simulink model "Slx001_Examine2_MHMP"  (R2017b)
settings: Solver=FixedStepAuto  StartTime=0.0  StopTime=100  FixedStep=0.1  RelTol=1e-3
libraries: neural x203
(part 3 of 3)

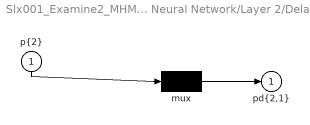
== system Slx001_Examine2_MHMP/Custom Neural Network/Layer 2/Delays 1 ==
  "p{2}" : Inport  PortDimensions=200
      mask Display: e = 0.06;c1 = [120 230 180]/255;c2 = ([120 230 180]+0)/(256+128);c3 = ([120 230 180]+128)/(256+128);patch([0 1 1 0],[0 0 1 1],c1);patch([0 1 1 1-e 1-e 0+e],[0 0 1 1-e 0+e 0+e],c2);patch([0 0 1 1-e 0+e 0+e],[0 1 1 1-e 1-e 0+e],c3);plot([0 1 1 0 0],[0 0 1 1 0]);
  mux : Mux  Inputs=1
      mask Display: e = 0.06;c1 = [120 150 230]/255;c2 = ([120 150 230]+0)/383;c3 = ([120 150 230]+128)/383;patch([0 1 1 0],[0 0 1 1],c1);patch([0 1 1 1-e 1-e 0+e],[0 0 1 1-e 0+e 0+e],c2);patch([0 0 1 1-e 0+e 0+e],[0 1 1 1-e 1-e 0+e],c3);plot([0 1 1 0 0],[0 0 1 1 0]);disp('Mux')
  "pd{2,1}" : Outport
      mask Display: e = 0.06;c1 = [120 230 180]/255;c2 = ([120 230 180]+0)/(256+128);c3 = ([120 230 180]+128)/(256+128);patch([0 1 1 0],[0 0 1 1],c1);patch([0 1 1 1-e 1-e 0+e],[0 0 1 1-e 0+e 0+e],c2);patch([0 0 1 1-e 0+e 0+e],[0 1 1 1-e 1-e 0+e],c3);plot([0 1 1 0 0],[0 0 1 1 0]);
  wires:
  "p{2}"/1 -> mux/1
  mux/1 -> "pd{2,1}"/1

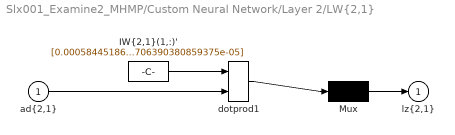
== system Slx001_Examine2_MHMP/Custom Neural Network/Layer 2/LW{2,1} ==
  "ad{2,1}" : Inport  PortDimensions=200
      mask Display: e = 0.06;c1 = [120 230 180]/255;c2 = ([120 230 180]+0)/(256+128);c3 = ([120 230 180]+128)/(256+128);patch([0 1 1 0],[0 0 1 1],c1);patch([0 1 1 1-e 1-e 0+e],[0 0 1 1-e 0+e 0+e],c2);patch([0 0 1 1-e 0+e 0+e],[0 1 1 1-e 1-e 0+e],c3);plot([0 1 1 0 0],[0 0 1 1 0]);
  "IW{2,1}(1,:)'" : Constant  Value=[0.00058445186548267678318391293856848278664983808994293212890625;0.0002747261203061034974537424346863190294243395328521728515625;-0.030217743541767448645085636371732107363641262054443359375;-1.23963834057929123133590110228396952152252197265625;-1.2698476867756418595689638095791451632976531982421875;0.00085237823747272810359643102628979249857366085052490234375;0.04076422815964921009257437845008098520338535308837890625;4.1971893208614599046768489643000066280364990234375;-4.0944749782750005095977030578069388866424560546875;-0.06225968966805582593959655923754326067864894866943359375;-0.0011034634817245103817484608299537285347469151020050048828125;-0.000501167222623257672779739646529151286813430488109588623046875;0.0011662017799871915446630055157584138214588165283203125;5.25253357376225249453227661433629691600799560546875;2.235674736283797425784314327756874263286590576171875;-3.01469607940744399598997915745712816715240478515625;1.0980579469144162718663437772192992269992828369140625;-1.097784902459118416828687259112484753131866455078125;-1.1895564096614303917220922812703065574169158935546875;1.1904110614466263395883061093627475202083587646484375;1.22650427450624821545943632372654974460601806640625;1.227256246488297453112181756296195089817047119140625;-1.2636508060369688877244698232971131801605224609375;-1.26374426363649394744470555451698601245880126953125;-0.43725143683479072986841629244736395776271820068359375;-4.8554689277195084429195048869587481021881103515625;-4.41455355940285709692716409335844218730926513671875;-3.3362760558282378298144976724870502948760986328125;-2.468238247988046918379723138059489428997039794921875;5.80921865827347172483996473602019250392913818359375;-0.001428905042815085089935589479637201293371617794036865234375;1.8116735249189961365345880039967596530914306640625;-1.8203056285913230549766694821300916373729705810546875;2.70300892386619384666346377343870699405670166015625;-2.71561855412486874428168448503129184246063232421875;-0.006285092353715431012783909636709722690284252166748046875;2.0027856574846598647354767308570444583892822265625;-6.92306960540523874669815995730459690093994140625;-4.915149258245431695968363783322274684906005859375;-2.738413499114486615582109152455814182758331298828125;2.748877401575802625899314080015756189823150634765625;-0.009302208628810114399154684861059649847447872161865234375;-3.169613434164340493026656986330635845661163330078125;3.191994234881607273024428650387562811374664306640625;2.74816549537731358299197381711564958095550537109375;2.727954706335268486583345293183811008930206298828125;2.72605861001428451118044904433190822601318359375;-2.73835721891323036203402807586826384067535400390625;-0.0183380419939061685419279257303060148842632770538330078125;2.846837303777656646985860788845457136631011962890625;2.8573113528761240331732551567256450653076171875;-0.007529266892117991195887416466803188086487352848052978515625;-2.3511064355942767889473543618805706501007080078125;2.35986804710449948885297999368049204349517822265625;-0.0129788157014909984188211211630914476700127124786376953125;3.04555538078304977034349576570093631744384765625;-3.056624435655217464358202050789259374141693115234375;-1.5949145159982041075608094615745358169078826904296875;-1.597647075316071418882302168640308082103729248046875;-1.9444539043328854521774928798549808561801910400390625;1.95007979158207067627017750055529177188873291015625;-2.587142001746624231373061775229871273040771484375;-2.597662994669156066862569787190295755863189697265625;-0.0121517937621135295456209490794208250008523464202880859375;-3.307601674130053570621612379909493029117584228515625;-3.32147640426576185035401067580096423625946044921875;0.01469283705233643232135332112875403254292905330657958984375;-3.095232759354845430976865827688015997409820556640625;-3.10750182200160285361789647140540182590484619140625;0.011470410027950080078529282445742865093052387237548828125;2.513148144753169166421002955758012831211090087890625 ...(+7297 chars)]
      mask Display: e = 0.06;c1 = [120 150 230]/255;c2 = ([120 150 230]+0)/383;c3 = ([120 150 230]+128)/383;patch([0 1 1 0],[0 0 1 1],c1);patch([0 1 1 1-e 1-e 0+e],[0 0 1 1-e 0+e 0+e],c2);patch([0 0 1 1-e 0+e 0+e],[0 1 1 1-e 1-e 0+e],c3);plot([0 1 1 0 0],[0 0 1 1 0]);disp('weights');
  Mux : Mux  Inputs=1
      mask Display: e = 0.06;c1 = [120 150 230]/255;c2 = ([120 150 230]+0)/383;c3 = ([120 150 230]+128)/383;patch([0 1 1 0],[0 0 1 1],c1);patch([0 1 1 1-e 1-e 0+e],[0 0 1 1-e 0+e 0+e],c2);patch([0 0 1 1-e 0+e 0+e],[0 1 1 1-e 1-e 0+e],c3);plot([0 1 1 0 0],[0 0 1 1 0]);disp('Mux');
  dotprod1 : neural/Weight Functions/dotprod
  "lz{2,1}" : Outport
      mask Display: e = 0.06;c1 = [120 230 180]/255;c2 = ([120 230 180]+0)/(256+128);c3 = ([120 230 180]+128)/(256+128);patch([0 1 1 0],[0 0 1 1],c1);patch([0 1 1 1-e 1-e 0+e],[0 0 1 1-e 0+e 0+e],c2);patch([0 0 1 1-e 0+e 0+e],[0 1 1 1-e 1-e 0+e],c3);plot([0 1 1 0 0],[0 0 1 1 0]);
  wires:
  "IW{2,1}(1,:)'"/1 -> dotprod1/1
  "ad{2,1}"/1 -> dotprod1/2
  dotprod1/1 -> Mux/1
  Mux/1 -> "lz{2,1}"/1

== matlab function Slx001_Examine2_MHMP/MATLAB Function1 ==
  data: x input; y output
function y = fcn(x)
C = [1 0 0 0;
     0 1 0 0;
     0 0 1 0;
     0 0 0 1];
D = 0;
y = C*x + D;

== matlab function Slx001_Examine2_MHMP/MATLAB Function ==
  data: x input; u input; x_dot output
function x_dot = fcn(x, u)
K1=5; K2=7; D1=40; D2=30; M1=2; M2=3;

A = [0 1 0 0;
    -K2/M2 -D2/M2 K1/M2 D1/M2;
    0 0 0 1
    (K1-K2)/M1 (D1-D2)/M1 -K1/M1 -D1/M1];

B = [0; 0; 0; 1/M1];
x_dot = A*x + B*u;
